simulink model "Initiate_simulation"  (R2023a)
settings: Solver=VariableStepAuto  StartTime=0.0  StopTime=Inf  RelTol=1e-3
undefined symbols (not defined in the file or in its folder): max_deflections
libraries: aerolibanimutils x2, arduinolib x1, FlightInstruments x1, FlightSimulation_FlightMechanics_LibModelModified x1, SimulinkToXPlane11 x1
settings Model: Creator=setup  LastModifiedBy=LSV-PC0
settings DataIOCC: SaveState=on
settings DebuggingCC: UnconnectedInputMsg=warning  UnconnectedOutputMsg=warning  UnconnectedLineMsg=warning
settings ModelReferenceCC: EnableRefExpFcnMdlSchedulingChecks=on
settings RTWCC: DLArmComputeVersion=19.05

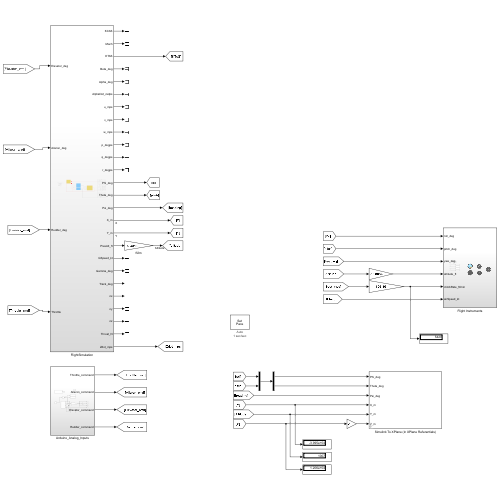
[thumbnail: Simulink's stored preview of the top-level diagram]
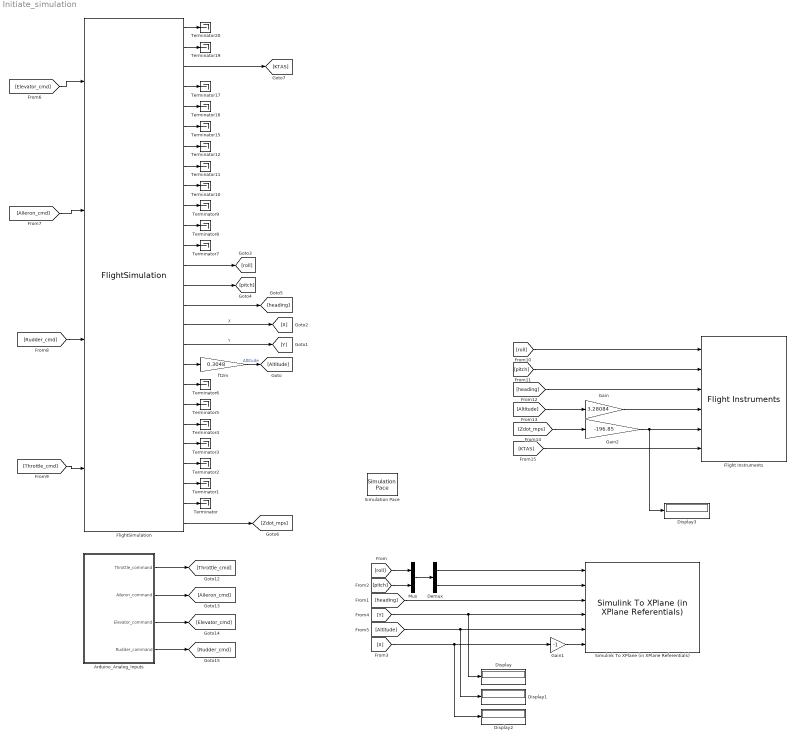
== system Initiate_simulation ==
  Arduino_Analog_Inputs : Subsystem
  Demux : Demux  Outputs=2
  Display{,1..3} (4 alike) : Display
  Flight Instruments : FlightInstruments/Flight Instruments  SystemSampleTime=-1  VariantActivationTime=update diagram  Latency=0  AutoFrameSizeCalculation=off
  FlightSimulation : FlightSimulation_FlightMechanics_LibModelModified/FlightSimulation  SystemSampleTime=-1  VariantActivationTime=update diagram  Latency=0  AutoFrameSizeCalculation=off
  Gain : Gain  Gain=3.28084
  Gain1 : Gain  Gain=-1
  Gain2 : Gain  Gain=-196.85
  Mux : Mux  Inputs=2
  Simulation Pace : aerolibanimutils/Simulation Pace  SimulationPace=1  SleepMode=Auto  OutputPaceError=off  SampleTime=1/60
  Simulink To XPlane (in XPlane Referentials) : SimulinkToXPlane11/Simulink To XPlane (in XPlane Referentials)  Precision=5
  Terminator{,1..12,15..17,19..20} (18 alike) : Terminator
  ft2m : Gain  Gain=0.3048
  wires:
  FlightSimulation/18 -> ft2m/1
  ft2m/1 -> [Altitude]  "Altitude"
  FlightSimulation/17 -> [Y]  "Y"
  FlightSimulation/16 -> [X]  "X"
  FlightSimulation/25 -> Terminator/1
  FlightSimulation/24 -> Terminator1/1
  FlightSimulation/22 -> Terminator3/1
  FlightSimulation/23 -> Terminator2/1
  FlightSimulation/21 -> Terminator4/1
  FlightSimulation/19 -> Terminator6/1
  FlightSimulation/20 -> Terminator5/1
  FlightSimulation/9 -> Terminator10/1
  FlightSimulation/13 -> [roll]
  FlightSimulation/14 -> [pitch]
  FlightSimulation/15 -> [heading]
  FlightSimulation/1 -> Terminator20/1
  FlightSimulation/2 -> Terminator19/1
  FlightSimulation/3 -> [KTAS]
  FlightSimulation/4 -> Terminator17/1
  FlightSimulation/5 -> Terminator16/1
  FlightSimulation/6 -> Terminator15/1
  FlightSimulation/7 -> Terminator12/1
  FlightSimulation/8 -> Terminator11/1
  Arduino_Analog_Inputs/1(Throttle_command) -> [Throttle_cmd]
  Arduino_Analog_Inputs/2(Aileron_command) -> [Aileron_cmd]
  Arduino_Analog_Inputs/3(Elevator_command) -> [Elevator_cmd]
  Arduino_Analog_Inputs/4(Rudder_command) -> [Rudder_cmd]
  [Elevator_cmd] -> FlightSimulation/1
  [Aileron_cmd] -> FlightSimulation/2
  [Rudder_cmd] -> FlightSimulation/3
  [Throttle_cmd] -> FlightSimulation/4
  FlightSimulation/10 -> Terminator9/1
  FlightSimulation/11 -> Terminator8/1
  FlightSimulation/12 -> Terminator7/1
  [heading] -> Simulink To XPlane (in XPlane Referentials)/3
  [Y] -> Simulink To XPlane (in XPlane Referentials)/4, Display/1
  [Altitude] -> Simulink To XPlane (in XPlane Referentials)/5, Display1/1
  Gain1/1 -> Simulink To XPlane (in XPlane Referentials)/6
  [X] -> Display2/1, Gain1/1
  [pitch] -> Mux/2
  [roll] -> Mux/1
  Mux/1 -> Demux/1
  Demux/1 -> Simulink To XPlane (in XPlane Referentials)/1
  Demux/2 -> Simulink To XPlane (in XPlane Referentials)/2
  [roll] -> Flight Instruments/1
  [pitch] -> Flight Instruments/2
  [heading] -> Flight Instruments/3
  Gain/1 -> Flight Instruments/4
  [Altitude] -> Gain/1
  FlightSimulation/26 -> [Zdot_mps]
  Gain2/1 -> Flight Instruments/5, Display3/1
  [Zdot_mps] -> Gain2/1
  [KTAS] -> Flight Instruments/6

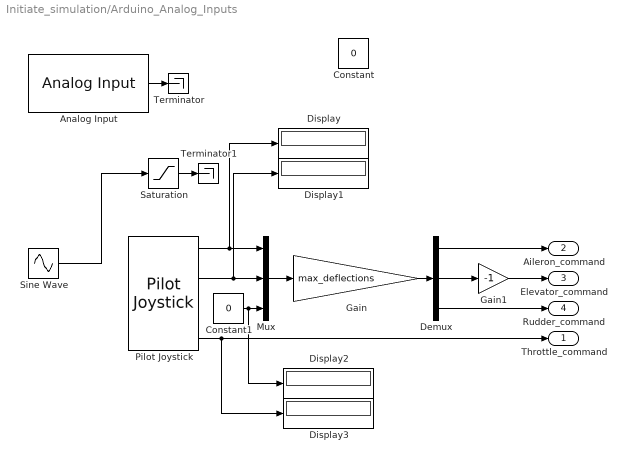
== system Initiate_simulation/Arduino_Analog_Inputs ==
  Analog Input : arduinolib/Analog Input  pinNumber=4  ReadResultsOnly=off  ConversionTriggerSource=Software  ExternalTriggerType=uint32( 0 )  OutputDataType=uint16  EnableConversionCompleteNotify=off  EnableOuputStatus=off  SampleTime=-1  blockPlatform=arduino
  Constant : Constant  Value=0
  Constant1 : Constant  Value=0
  Demux : Demux  Outputs=3
  Display{,1..3} (4 alike) : Display
  Gain : Gain  Gain=max_deflections  OutMin=-3  OutMax=5
  Gain1 : Gain  Gain=-1
  Mux : Mux  Inputs=3
  Pilot Joystick : aerolibanimutils/Pilot Joystick  JoystickID=Joystick1  OutputConfiguration=FourAxis  SampleTime=1/60
  Saturation : Saturate  UpperLimit=1  LowerLimit=0
  Sine Wave : Sin  SampleTime=0
  Terminator : Terminator
  Terminator1 : Terminator
  Throttle_command : Outport
  Aileron_command : Outport  Port=2
  Elevator_command : Outport  Port=3
  Rudder_command : Outport  Port=4
  wires:
  Sine Wave/1 -> Saturation/1
  Analog Input/1 -> Terminator/1
  Saturation/1 -> Terminator1/1
  Pilot Joystick/1 -> Display/1, Mux/1
  Pilot Joystick/2 -> Display1/1, Mux/2
  Pilot Joystick/4 -> Display3/1, Throttle_command/1
  Mux/1 -> Gain/1
  Gain/1 -> Demux/1
  Demux/1 -> Aileron_command/1
  Demux/3 -> Rudder_command/1
  Constant1/1 -> Display2/1, Mux/3
  Demux/2 -> Gain1/1
  Gain1/1 -> Elevator_command/1
